simulink model "MIEM_Adaptive"  (Simulink 7.8)
settings: Solver=ode1  StartTime=0.0  StopTime=inf  FixedStep=0.001  RelTol=1e-3
undefined symbols (not defined in the file): HIL, qc_get_step_size
libraries: quarc_library x39, simulink x20, dspmtrx3 x3
(part 2 of 2)

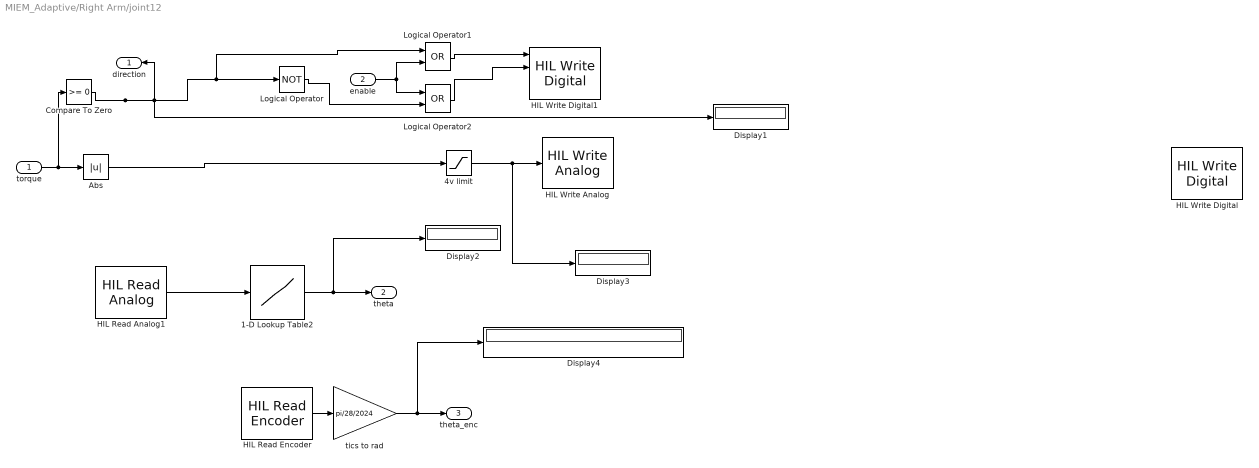
== system MIEM_Adaptive/Right Arm/joint12 ==
  torque : Inport
  enable : Inport  Port=2
  1-D Lookup Table2 : Lookup_n-D  NumberOfTableDimensions=1  BreakpointsForDimension1=[.78 1.64 2.51 3.40 4.27]  Table=[2 1 0 -1 -2]  RndMeth=Simplest  InputSameDT=on
  4v limit : Saturate  UpperLimit=4  LowerLimit=0
  Abs : Abs
  Compare To Zero : simulink/Logic and Bit Operations/Compare To Zero  relop=>=  OutDataTypeStr=boolean
  Display{1..4} (4 alike) : Display
  HIL Read Analog1 : quarc_library/Data Acquisition/Generic/Immediate I//O/HIL Read Analog  object_name=HIL-1  channels=[3]  sample_time=qc_get_step_size  active=on  vector_output=off
  HIL Read Encoder : quarc_library/Data Acquisition/Generic/Immediate I//O/HIL Read Encoder  object_name=HIL-2  channels=[1]  sample_time=qc_get_step_size  active=on  vector_output=off  data_type_mode=Inherit via back propagation  data_type=double
  HIL Write Analog : quarc_library/Data Acquisition/Generic/Immediate I//O/HIL Write Analog  object_name=HIL-1  channels=[1]  sample_time=-1  active=off  vector_input=off
  HIL Write Digital : quarc_library/Data Acquisition/Generic/Immediate I//O/HIL Write Digital  object_name=HIL-1  channels=[4:7]  sample_time=-1  active=off  vector_input=off
  HIL Write Digital1 : quarc_library/Data Acquisition/Generic/Immediate I//O/HIL Write Digital  object_name=HIL-1  channels=[44:47]  sample_time=-1  active=off  vector_input=off
  Logical Operator : Logic  Operator=NOT  AllPortsSameDT=off  OutDataTypeStr=boolean
  Logical Operator1 : Logic  Operator=OR  AllPortsSameDT=off  OutDataTypeStr=boolean
  Logical Operator2 : Logic  Operator=OR  AllPortsSameDT=off  OutDataTypeStr=boolean
  tics to rad : Gain  Gain=pi/28/2024
  direction : Outport
  theta : Outport  Port=2
  theta_enc : Outport  Port=3
  wires:
  4v limit/1 -> HIL Write Analog/1, Display3/1
  Compare To Zero/1 -> Logical Operator/1, Logical Operator1/1, direction/1, Display1/1
  Abs/1 -> 4v limit/1
  torque/1 -> Abs/1, Compare To Zero/1
  HIL Read Analog1/1 -> 1-D Lookup Table2/1
  HIL Read Encoder/1 -> tics to rad/1
  Logical Operator1/1 -> HIL Write Digital1/1
  Logical Operator2/1 -> HIL Write Digital1/2
  Logical Operator/1 -> Logical Operator2/2
  enable/1 -> Logical Operator1/2, Logical Operator2/1
  tics to rad/1 -> theta_enc/1, Display4/1
  1-D Lookup Table2/1 -> Display2/1, theta/1

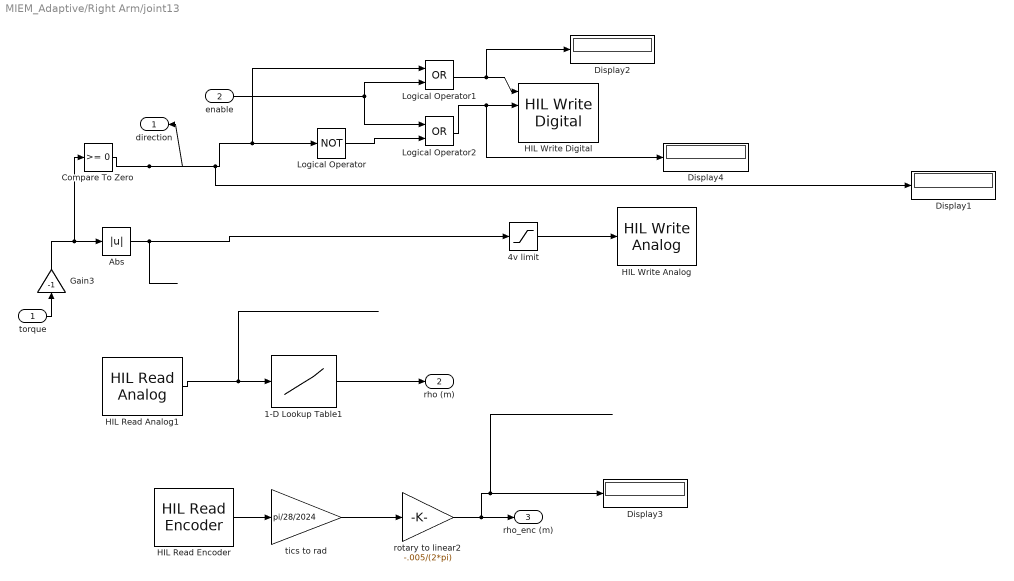
== system MIEM_Adaptive/Right Arm/joint13 ==
  torque : Inport
  enable : Inport  Port=2
  1-D Lookup Table1 : Lookup_n-D  NumberOfTableDimensions=1  BreakpointsForDimension1="[.255 .369 .511 .661 .806 .966 1.075  1.274 1.456 1.643 1.858 2.075 2.328 2.50 2.753 3.011 3.23 3.39 4 4.191 4.384 4.628 4.84 4.963]"  Table=[0 .004 .0067 .0094 .012 .015 .017 .0199 .022 .0245 .0263 .0279 .0287 .0294 .030 .0315 .032 .034 .0357 .0365 .0373 .0385 .039 .04]+.001  RndMeth=Simplest  InputSameDT=on
  4v limit : Saturate  UpperLimit=4  LowerLimit=0
  Abs : Abs
  Compare To Zero : simulink/Logic and Bit Operations/Compare To Zero  relop=>=  OutDataTypeStr=boolean
  Display{1..4} (4 alike) : Display
  Gain3 : Gain  Gain=-1
  HIL Read Analog1 : quarc_library/Data Acquisition/Generic/Immediate I//O/HIL Read Analog  object_name=HIL-2  channels=[5]  sample_time=qc_get_step_size  active=on  vector_output=off
  HIL Read Encoder : quarc_library/Data Acquisition/Generic/Immediate I//O/HIL Read Encoder  object_name=HIL-2  channels=[2]  sample_time=qc_get_step_size  active=on  vector_output=off  data_type_mode=Inherit via back propagation  data_type=double
  HIL Write Analog : quarc_library/Data Acquisition/Generic/Immediate I//O/HIL Write Analog  object_name=HIL-1  channels=[2]  sample_time=-1  active=off  vector_input=off
  HIL Write Digital : quarc_library/Data Acquisition/Generic/Immediate I//O/HIL Write Digital  object_name=HIL-1  channels=[8:11]  sample_time=-1  active=off  vector_input=off
  Logical Operator : Logic  Operator=NOT  AllPortsSameDT=off  OutDataTypeStr=boolean
  Logical Operator1 : Logic  Operator=OR  AllPortsSameDT=off  OutDataTypeStr=boolean
  Logical Operator2 : Logic  Operator=OR  AllPortsSameDT=off  OutDataTypeStr=boolean
  rotary to linear2 : Gain  Gain=-.005/(2*pi)
  tics to rad : Gain  Gain=pi/28/2024
  direction : Outport
  rho (m) : Outport  Port=2
  rho_enc (m) : Outport  Port=3
  wires:
  4v limit/1 -> HIL Write Analog/1
  Compare To Zero/1 -> Logical Operator/1, Logical Operator1/1, Display1/1, direction/1
  Abs/1 -> 4v limit/1
  torque/1 -> Gain3/1
  HIL Read Analog1/1 -> 1-D Lookup Table1/1
  HIL Read Encoder/1 -> tics to rad/1
  Logical Operator/1 -> Logical Operator2/2
  Logical Operator2/1 -> HIL Write Digital/2, Display4/1
  Logical Operator1/1 -> HIL Write Digital/1, Display2/1
  enable/1 -> Logical Operator1/2, Logical Operator2/1
  1-D Lookup Table1/1 -> rho (m)/1
  tics to rad/1 -> rotary to linear2/1
  rotary to linear2/1 -> rho_enc (m)/1, Display3/1
  Gain3/1 -> Abs/1, Compare To Zero/1

== system MIEM_Adaptive/IK_L/phantom/haptic gravity compensation ==
  position : Inport
  boundary force : Inport  Port=2
  Constant : Constant  Value=[0 0 .92]
  Derivative : Derivative
  Derivative1 : Derivative
  Gain : Gain  Gain=-2*diag([1 1 1])  Multiplication=Matrix(K*u)
  Gain1 : Gain  Gain=-0e-2*diag([1 1 1])  Multiplication=Matrix(K*u)
  Gain2 : Gain  Gain=-4*diag([1 1 1])  Multiplication=Matrix(K*u)
  Saturation : Saturate  UpperLimit=3  LowerLimit=-3
  Sum : Sum  Inputs=|+++++
  force : Outport
  wires:
  Gain/1 -> Sum/2
  Derivative/1 -> Gain/1, Derivative1/1, Gain2/1
  Derivative1/1 -> Gain1/1
  Gain1/1 -> Sum/1
  Sum/1 -> Saturation/1
  position/1 -> Derivative/1
  Saturation/1 -> force/1
  boundary force/1 -> Sum/5
  Constant/1 -> Sum/4
  Gain2/1 -> ?

== matlab function Left Arm/controller 24/slotine's adaptive ==
  data: en input double; lambda input double; gamma input double; qd input double; qddot input double; qddotdot input double; q input double; tau output double; qdot input double; ahat output double; ahat_ input double
function [tau,ahat] = fcn(en,lambda,gamma,qd,qddot,qddotdot,q,qdot,ahat_)
%#codegen


qtilde=q-qd;
qtildedot=qdot-qddot;
s=qtildedot+lambda*qtilde;
Y=[qddotdot qddot sign(qdot) s ];
ahat=-.001*en/gamma*Y'*s+ahat_;
qr=qd-(ahat(end)+lambda)*qtilde;
qrdot=qddot-(ahat(end)+lambda)*qtilde;
qrdotdot=qddotdot-(ahat(end)+lambda)*qtildedot;

tau=[qrdotdot qrdot  sign(qdot) s ]*ahat;

== matlab function scheduler/scheduler ==
  data: status_ input double; qd0_L_ input double; qd0_R_ input double; qpot_L input double; qpot_R input double; qenc_L input double; qenc_R input double; time input double; status output double; qd0_L output double; qd0_R output double; ready output double; ready_ input double; delq_L_ input double; delq_L output double; delq_R_ input double; delq_R output double
function [status,qd0_L,qd0_R,ready,delq_L,delq_R]  = fcn(status_,qd0_L_,qd0_R_,qpot_L,qpot_R,qenc_L,qenc_R,time,ready_,delq_L_,delq_R_)
%#codegen
status=status_;
ready=ready_;
qd0_L=qd0_L_;
qd0_R=qd0_R_;

if time<=.1
    delq_L=qpot_L;
    delq_R=qpot_R;
else
    delq_L=delq_L_;
    delq_R=delq_R_;
end

%first wait for 1 sec

if time>5 && not(ready)
    
    switch status
        case 0
            %check left arm joit 2
            if abs(qpot_L(2))<.1
                %left arm joint 2 home already
                status=1;
            else
                %home left arm joint 2
                qd0_L=-[0 delq_L(2) 0 0]';
            end
        case 1
            if abs(qpot_L(1))<.001 && time>8
                %left arm joint 1 home already
                status=2;
            else
                %left arm home joint 1
                qd0_L=-[delq_L(1) delq_L(2) 0 0]';
            end
        case 2
            if abs(qpot_L(3))<.001 && time>12
                %left arm joint 2 home already
                status=3;
            else
                %left arm home joint 2
                qd0_L=-[delq_L(1) delq_L(2) delq_L(3) 0]';
            end
        case 3
            %check right arm joit 2
            if abs(qpot_R(2))<.1 && time>16
                %right arm joint 2 home already
                status=4;
            else
                %home left arm joint 2
                qd0_R=-[0 delq_R(2) 0 0]';
            end
        case 4
            if abs(qpot_R(1))<.001 && time>20
                %right arm joint 1 home already
                status=5;
            else
                %right arm home joint 1
                qd0_R=-[delq_R(1) delq_R(2) 0 0]';
            end
        case 5
            if abs(qpot_R(3))<.001 && time>24
                %right arm joint 2 home already
                status=6;
            else
                %right arm home joint 2
                qd0_R=-[delq_R(1) delq_R(2) delq_R(3) 0]';
            end

        case 6
            qd0_L=-[delq_L(1) delq_L(2) delq_L(3) 0]';
            qd0_R=-[delq_R(1) delq_R(2) delq_R(3) 0]';
            ready=1;
    end
    
    
end

== matlab function filter/filter ==
  data: u input double; y output double; u_ input double
function y = fcn(u,u_)
%#codegen
if u>0
    a=2;
end
if abs(u-u_)<4*pi*.001
    y=u;
else
    y=u_+4*pi*.001*(u-u_)/abs(u-u_);

end

== matlab function Left Arm/controller 23/slotine's adaptive ==
  data: en input double; lambda input double; gamma input double; qd input double; qddot input double; qddotdot input double; q input double; tau output double; qdot input double; ahat output double; ahat_ input double
function [tau,ahat] = fcn(en,lambda,gamma,qd,qddot,qddotdot,q,qdot,ahat_)
%#codegen


qtilde=q-qd;
qtildedot=qdot-qddot;
s=qtildedot+lambda*qtilde;
Y=[qddotdot qddot sign(qdot) s ];
ahat=-.001*en/gamma*Y'*s+ahat_;
qr=qd-(ahat(end)+lambda)*qtilde;
qrdot=qddot-(ahat(end)+lambda)*qtilde;
qrdotdot=qddotdot-(ahat(end)+lambda)*qtildedot;

tau=[qrdotdot qrdot  sign(qdot) s ]*ahat;

== matlab function filter1/filter ==
  data: u input double; y output double; u_ input double
function y = fcn(u,u_)
%#codegen
if u>0
    a=2;
end
if abs(u-u_)<.02*.001
    y=u;
else
    y=u_+.02*.001*(u-u_)/abs(u-u_);

end

== matlab function Left Arm/contoller 22/slotine's adaptive ==
  data: en input double; lambda input double; gamma input double; qd input double; qddot input double; qddotdot input double; q input double; tau output double; qdot input double; ahat output double; ahat_ input double
function [tau,ahat] = fcn(en,lambda,gamma,qd,qddot,qddotdot,q,qdot,ahat_)
%#codegen


qtilde=q-qd;
qtildedot=qdot-qddot;
s=qtildedot+lambda*qtilde;
Y=[qddotdot qddot sign(qdot) s ];
ahat=-.001*en/gamma*Y'*s+ahat_;
qr=qd-(ahat(end)+lambda)*qtilde;
qrdot=qddot-(ahat(end)+lambda)*qtilde;
qrdotdot=qddotdot-(ahat(end)+lambda)*qtildedot;

tau=[qrdotdot qrdot  sign(qdot) s ]*ahat;

== matlab function filter2/filter ==
  data: u input double; y output double; u_ input double
function y = fcn(u,u_)
%#codegen
if u>0
    a=2;
end
if abs(u-u_)<4*pi*.001
    y=u;
else
    y=u_+4*pi*.001*(u-u_)/abs(u-u_);

end

== matlab function Left Arm/controller 21/slotine's adaptive ==
  data: en input double; lambda input double; gamma input double; qd input double; qddot input double; qddotdot input double; q input double; tau output double; qdot input double; ahat output double; ahat_ input double
function [tau,ahat] = fcn(en,lambda,gamma,qd,qddot,qddotdot,q,qdot,ahat_)
%#codegen


qtilde=q-qd;
qtildedot=qdot-qddot;
s=qtildedot+lambda*qtilde;
Y=[qddotdot qddot  sign(qdot)-1 sign(qdot)+1 s ];
ahat=-.001*en/gamma*Y'*s+ahat_;
qr=qd-(ahat(end)+lambda)*qtilde;
qrdot=qddot-(ahat(end)+lambda)*qtilde;
qrdotdot=qddotdot-(ahat(end)+lambda)*qtildedot;

tau=[qrdotdot qrdot sign(qdot)-1 sign(qdot)+1 s ]*ahat;

== matlab function filter3/filter ==
  data: u input double; y output double; u_ input double
function y = fcn(u,u_)
%#codegen
if u>0
    a=2;
end
if abs(u-u_)<.02*.001
    y=u;
else
    y=u_+.02*.001*(u-u_)/abs(u-u_);

end

== matlab function Right Arm/contoller 22/slotine's adaptive ==
  data: en input double; lambda input double; gamma input double; qd input double; qddot input double; qddotdot input double; q input double; tau output double; qdot input double; ahat output double; ahat_ input double
function [tau,ahat] = fcn(en,lambda,gamma,qd,qddot,qddotdot,q,qdot,ahat_)
%#codegen


qtilde=q-qd;
qtildedot=qdot-qddot;
s=qtildedot+lambda*qtilde;
Y=[qddotdot qddot sign(qdot) s ];
ahat=-.001*en/gamma*Y'*s+ahat_;
qr=qd-(ahat(end)+lambda)*qtilde;
qrdot=qddot-(ahat(end)+lambda)*qtilde;
qrdotdot=qddotdot-(ahat(end)+lambda)*qtildedot;

tau=[qrdotdot qrdot  sign(qdot) s ]*ahat;

== matlab function IK_L/IK_L/IK ==
  data: q_ input double; q output double; qm output double; qdot output double; error output double; pd input double; pd_d input double; F output double; k_ input double; k output double; r_ input double; r output double
function [q,qm,qdot,error,F,k,r] = fcn(q_,pd,pd_d,k_,r_)
%#codegen
kappa=1/5;
x=pd(1);
y=pd(2);
z=pd(3);
r=sqrt(x^2+y^2);

rho_1=q_(1);
theta_1=q_(2);
rho_2=q_(3);
%%%%%
J =...
    [ -kappa*cos(kappa*rho_1)*cos(theta_1)*(rho_1 - (rho_2+1)),   (sin(theta_1)*(cos(kappa*rho_1) - 1))/kappa + sin(kappa*rho_1)*sin(theta_1)*(rho_1 - (rho_2+1)), sin(kappa*rho_1)*cos(theta_1)
    -kappa*cos(kappa*rho_1)*sin(theta_1)*(rho_1 - (rho_2+1)), - (cos(theta_1)*(cos(kappa*rho_1) - 1))/kappa - sin(kappa*rho_1)*cos(theta_1)*(rho_1 - (rho_2+1)), sin(kappa*rho_1)*sin(theta_1)
    kappa*sin(kappa*rho_1)*(rho_1 - (rho_2+1)),                                                                                             0,              cos(kappa*rho_1)];


qdot=pinv(J)*pd_d;

%IK
theta_1_=theta_1;
theta_1=atan2(y,x);

if theta_1-theta_1_>3*pi/2
    k=k_-1;
elseif theta_1_-theta_1>3*pi/2
    k=k_+1;
else
    k=k_;
end
    
del=sqrt(abs(((1-kappa*sqrt(x^2+y^2))^2+kappa^2*z^2-1)/kappa^2));%del=rho_2-rho_1
rho_1=1/kappa*atan2(-(-kappa*z-(1-kappa*r)*kappa*-del),-kappa^2*z*-del+(1-kappa*r));
rho_2=rho_1+del-1;


if rho_2>=4
    rho_2=4;
elseif rho_2<=.1
    rho_2=.1;
end

if rho_2-rho_1<=0.1
    rho_1=rho_2-0.1;
end
if rho_1<=.1
    rho_1=.1;
end



q=[rho_1;theta_1;rho_2];
qm=[rho_1;theta_1+2*k*pi;rho_2];



% J_ =...
%     [ -kappa*cos(kappa*rho_1)*cos(theta_1)*(rho_1 - (rho_2+1)),   (sin(theta_1)*(cos(kappa*rho_1) - 1))/kappa + sin(kappa*rho_1)*sin(theta_1)*(rho_1 - (rho_2+1)), sin(kappa*rho_1)*cos(theta_1), 0
%     -kappa*cos(kappa*rho_1)*sin(theta_1)*(rho_1 - (rho_2+1)), - (cos(theta_1)*(cos(kappa*rho_1) - 1))/kappa - sin(kappa*rho_1)*cos(theta_1)*(rho_1 - (rho_2+1)), sin(kappa*rho_1)*sin(theta_1), 0
%     kappa*sin(kappa*rho_1)*(rho_1 - (rho_2+1)),                                                                                             0,              cos(kappa*rho_1), 0];




q=[rho_1;theta_1;rho_2];

p =...
    [ - (cos(theta_1)*(cos(kappa*rho_1) - 1))/kappa - sin(kappa*rho_1)*cos(theta_1)*(rho_1 - (rho_2+1))
    - (sin(theta_1)*(cos(kappa*rho_1) - 1))/kappa - sin(kappa*rho_1)*sin(theta_1)*(rho_1 - (rho_2+1))
    sin(kappa*rho_1)/kappa - cos(kappa*rho_1)*(rho_1 - (rho_2+1))];



error=norm(pd-p);



%Force field barrier method
F=[0 0 0]';

if kappa*z<1
    s=asin(kappa*z)/kappa;
    if r>.95*(1-cos(kappa*s))/kappa
        F=(-10*abs(r-.9*(1-cos(kappa*s))/kappa))*[cos(theta_1)*cos(kappa*s);sin(theta_1)*cos(kappa*s);-sin(kappa)*s];
    end
end



end

== matlab function Right Arm/controller 21/slotine's adaptive ==
  data: en input double; lambda input double; gamma input double; qd input double; qddot input double; qddotdot input double; q input double; tau output double; qdot input double; ahat output double; ahat_ input double
function [tau,ahat] = fcn(en,lambda,gamma,qd,qddot,qddotdot,q,qdot,ahat_)
%#codegen


qtilde=q-qd;
qtildedot=qdot-qddot;
s=qtildedot+lambda*qtilde;
Y=[qddotdot qddot  sign(qdot)-1 sign(qdot)+1 s ];
ahat=-.001*en/gamma*Y'*s+ahat_;
qr=qd-(ahat(end)+lambda)*qtilde;
qrdot=qddot-(ahat(end)+lambda)*qtilde;
qrdotdot=qddotdot-(ahat(end)+lambda)*qtildedot;

tau=[qrdotdot qrdot sign(qdot)-1 sign(qdot)+1 s ]*ahat;

== matlab function Right Arm/controller 23/slotine's adaptive ==
  data: en input double; lambda input double; gamma input double; qd input double; qddot input double; qddotdot input double; q input double; tau output double; qdot input double; ahat output double; ahat_ input double
function [tau,ahat] = fcn(en,lambda,gamma,qd,qddot,qddotdot,q,qdot,ahat_)
%#codegen


qtilde=q-qd;
qtildedot=qdot-qddot;
s=qtildedot+lambda*qtilde;
Y=[qddotdot qddot sign(qdot) s ];
ahat=-.001*en/gamma*Y'*s+ahat_;
qr=qd-(ahat(end)+lambda)*qtilde;
qrdot=qddot-(ahat(end)+lambda)*qtilde;
qrdotdot=qddotdot-(ahat(end)+lambda)*qtildedot;

tau=[qrdotdot qrdot  sign(qdot) s ]*ahat;

== matlab function Right Arm/controller 24/slotine's adaptive ==
  data: en input double; lambda input double; gamma input double; qd input double; qddot input double; qddotdot input double; q input double; tau output double; qdot input double; ahat output double; ahat_ input double
function [tau,ahat] = fcn(en,lambda,gamma,qd,qddot,qddotdot,q,qdot,ahat_)
%#codegen


qtilde=q-qd;
qtildedot=qdot-qddot;
s=qtildedot+lambda*qtilde;
Y=[qddotdot qddot sign(qdot) s ];
ahat=-.001*en/gamma*Y'*s+ahat_;
qr=qd-(ahat(end)+lambda)*qtilde;
qrdot=qddot-(ahat(end)+lambda)*qtilde;
qrdotdot=qddotdot-(ahat(end)+lambda)*qtildedot;

tau=[qrdotdot qrdot  sign(qdot) s ]*ahat;

== matlab function filter4/filter ==
  data: u input double; y output double; u_ input double
function y = fcn(u,u_)
%#codegen
if u>0
    a=2;
end
if abs(u-u_)<4*pi*.001
    y=u;
else
    y=u_+4*pi*.001*(u-u_)/abs(u-u_);

end

== matlab function filter5/filter ==
  data: u input double; y output double; u_ input double
function y = fcn(u,u_)
%#codegen
if u>0
    a=2;
end
if abs(u-u_)<.02*.001
    y=u;
else
    y=u_+.02*.001*(u-u_)/abs(u-u_);

end

== matlab function filter6/filter ==
  data: u input double; y output double; u_ input double
function y = fcn(u,u_)
%#codegen
if u>0
    a=2;
end
if abs(u-u_)<4*pi*.001
    y=u;
else
    y=u_+4*pi*.001*(u-u_)/abs(u-u_);

end

== matlab function filter7/filter ==
  data: u input double; y output double; u_ input double
function y = fcn(u,u_)
%#codegen
if u>0
    a=2;
end
if abs(u-u_)<.02*.001
    y=u;
else
    y=u_+.02*.001*(u-u_)/abs(u-u_);

end
